simulink model "submission"  (R2023a)
settings: Solver=VariableStepAuto  StartTime=0.0  StopTime=50  RelTol=1e-3
model workspace (MAT data in the model file):
  TargetFrequency_56 = 2100000000
  TargetFrequency_64 = 2100000000
  TargetPhaseNoise_56 = [-85 -125 -150 -180]
  TargetPhaseNoise_64 = [-85 -125 -150 -180]
  uniqueStringPll_56 = '52_8533'
  uniqueStringPll_64 = '16_5649'
libraries: commrandsrc3 x2, commsynccomp2 x1, dspfdesign x1
settings Model: Creator=Zonularity  LastModifiedBy=Zonularity

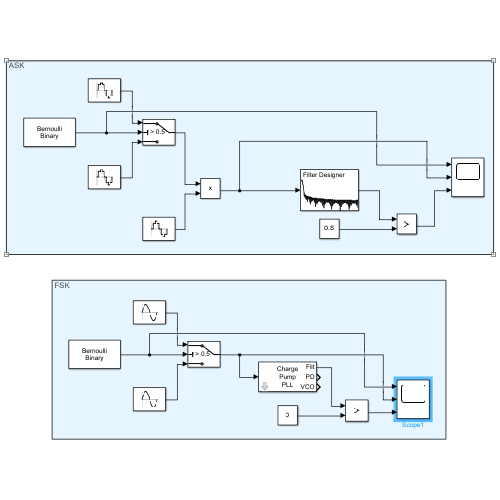
[thumbnail: Simulink's stored preview of the top-level diagram]
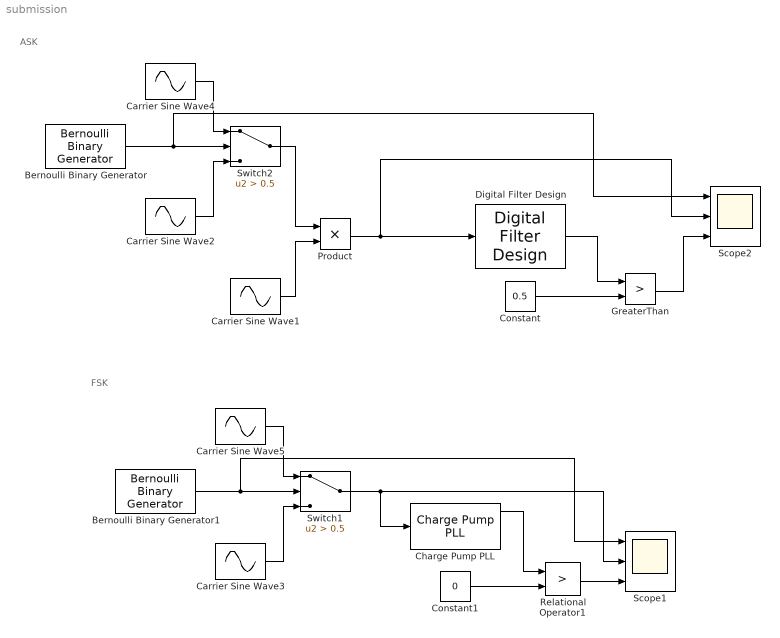
== system submission ==
  note: FSK
  note: ASK
  Bernoulli Binary Generator : commrandsrc3/Bernoulli Binary Generator  ProbabilityOfZero=0.5  SeedSource=Auto  Seed=0  SampleTime=1  SamplesPerFrame=1  OutputDataType=double  SimulateUsing=Interpreted execution
  Bernoulli Binary Generator1 : commrandsrc3/Bernoulli Binary Generator  ProbabilityOfZero=0.5  SeedSource=Auto  Seed=0  SampleTime=1  SamplesPerFrame=1  OutputDataType=double  SimulateUsing=Interpreted execution
  Carrier Sine Wave1 : Sin  Frequency=2*pi*4  SampleTime=0.01
  Carrier Sine Wave2 : Sin  Amplitude=0.5  Frequency=2*pi*4  SampleTime=0.01
  Carrier Sine Wave3 : Sin  Frequency=2*pi*4  SampleTime=0
  Carrier Sine Wave4 : Sin  Amplitude=2  Frequency=2*pi*4  SampleTime=0.01
  Carrier Sine Wave5 : Sin  Frequency=2*pi*12  SampleTime=0
  Charge Pump PLL : commsynccomp2/Charge Pump PLL  Fn=[2*pi*1]  Fd="[1   2*pi*1]"  Kvco=4  Fc=10  Ph=0  Ac=1
  Constant : Constant  Value=0.5
  Constant1 : Constant  Value=0
  Digital Filter Design : dspfdesign/Digital Filter Design  mwdsp_browser_bugfix_var=off
  GreaterThan : RelationalOperator  Operator=>  OutDataTypeStr=boolean  RndMeth=Simplest  InputSameDT=off
  Product : Product
  Relational Operator1 : RelationalOperator  Operator=>  OutDataTypeStr=boolean  RndMeth=Simplest  InputSameDT=off
  Scope1 : Scope  NumInputPorts=3
  Scope2 : Scope  NumInputPorts=3
  Switch1 : Switch  Criteria=u2 > Threshold  Threshold=0.5  SaturateOnIntegerOverflow=off  InputSameDT=off
  Switch2 : Switch  Criteria=u2 > Threshold  Threshold=0.5  SaturateOnIntegerOverflow=off  InputSameDT=off
  wires:
  Carrier Sine Wave3/1 -> Switch1/3
  Bernoulli Binary Generator1/1 -> Scope1/1, Switch1/2
  Carrier Sine Wave5/1 -> Switch1/1
  Constant1/1 -> Relational Operator1/2
  Charge Pump PLL/1 -> Relational Operator1/1
  Relational Operator1/1 -> Scope1/3
  Switch1/1 -> Scope1/2, Charge Pump PLL/1
  Switch2/1 -> Product/1
  Bernoulli Binary Generator/1 -> Scope2/1, Switch2/2
  Carrier Sine Wave4/1 -> Switch2/1
  Carrier Sine Wave1/1 -> Product/2
  Product/1 -> Scope2/2, Digital Filter Design/1
  Carrier Sine Wave2/1 -> Switch2/3
  Constant/1 -> GreaterThan/2
  Digital Filter Design/1 -> GreaterThan/1
  GreaterThan/1 -> Scope2/3
